simulink model "pcm_project"  (R2021b)
settings: Solver=VariableStepAuto  StartTime=0.0  StopTime=10  RelTol=1e-3
libraries: dspquant2 x2, dsparch4 x1, commutil2 x1, dspsigops x1
settings Model: Creator=ASUS i3  LastModifiedBy=ASUS i3
settings DataIOCC: SaveFormat=Array  SignalLoggingSaveFormat=ModelDataLogs  ReturnWorkspaceOutputs=off
settings OptimizationCC: BlockReduction=off  BooleanDataType=off
settings DebuggingCC: SaveWithParameterizedLinksMsg=none  UnderspecifiedInitializationDetection=Classic  MergeDetectMultiDrivingBlocksExec=none  SignalResolutionControl=TryResolveAllWithWarning  MultiTaskDSMMsg=warning  MultiTaskCondExecSysMsg=none  MultiTaskRateTransMsg=warning
settings HardwareCC: TargetUnknown=on
settings ModelReferenceCC: PropagateSignalLabelsOutOfModel=off
settings GRTTargetCC: CombineOutputUpdateFcns=off  GRTInterface=on

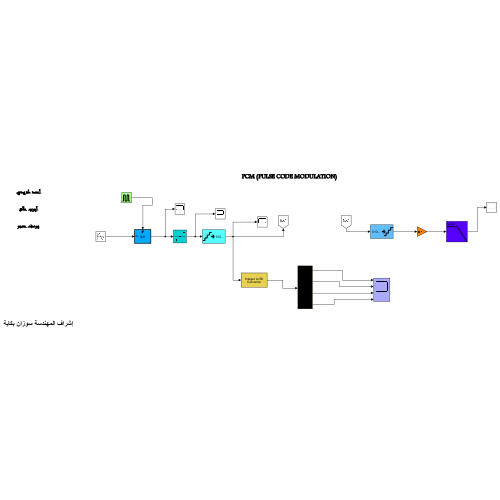
[thumbnail: Simulink's stored preview of the top-level diagram]
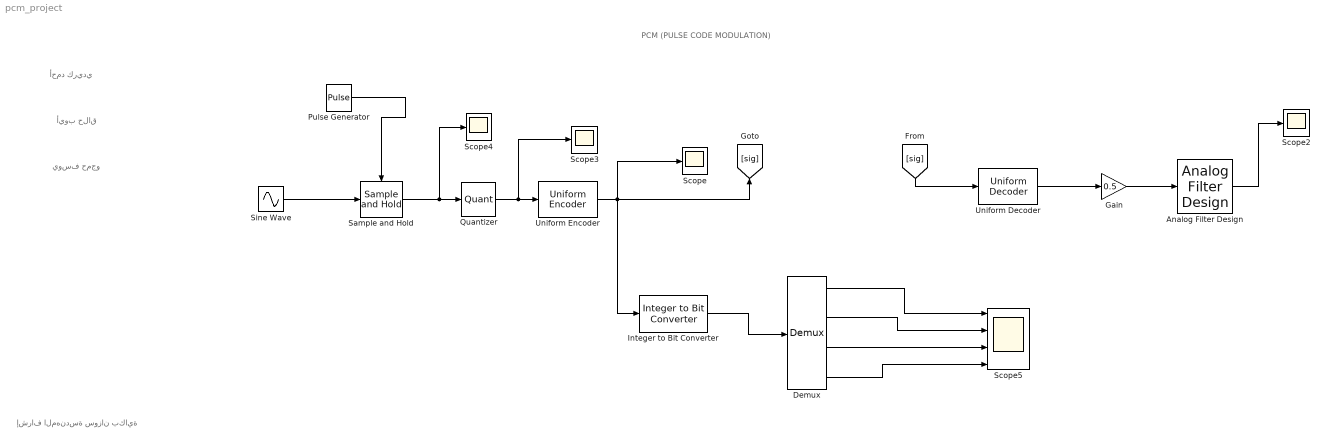
== system pcm_project ==
  note: يوسف حمجو
  note: أيوب حلاق
  note: أحمد كريدي
  note: إشراف المهندسة سوزان بكاية
  note: PCM (PULSE CODE MODULATION)
  Analog Filter Design : dsparch4/Analog Filter Design  method=Butterworth  filttype=Lowpass  N=8  Wlo=60  Whi=80  Rp=2  Rs=40
  Demux : Demux
  Gain : Gain  Gain=0.5
  Integer to Bit Converter : commutil2/Integer to Bit Converter  nbits=4  signedInputValues=Signed  bitOrder=MSB first  outDtype=Inherit via internal rule
  Pulse Generator : DiscretePulseGenerator  PulseType=Time based  Period=1/500  PulseWidth=5
  Quantizer : Quantizer  LinearizeAsGain=off
  Sample and Hold : dspsigops/Sample and Hold  trig=Rising edge  initCond=0  latchinput=off
  Scope{,2..4} (4 alike) : Scope
  Scope5 : Scope  NumInputPorts=4
  Sine Wave : Sin  Amplitude=5  Frequency=50  SampleTime=0
  Uniform Decoder : dspquant2/Uniform Decoder  peak=1  bits=3  overflowMode=Saturate  otype=Double
      settings: SourceProductBaseCode=DS
  Uniform Encoder : dspquant2/Uniform Encoder  peak=5  bits=4  otype=Signed integer
  wires:
  Sine Wave/1 -> Sample and Hold/1
  Sample and Hold/1 -> Scope4/1, Quantizer/1
  Uniform Encoder/1 -> Scope/1, [sig], Integer to Bit Converter/1
  Quantizer/1 -> Scope3/1, Uniform Encoder/1
  Integer to Bit Converter/1 -> Demux/1
  Demux/1 -> Scope5/1
  Demux/2 -> Scope5/2
  Demux/3 -> Scope5/3
  Demux/4 -> Scope5/4
  Uniform Decoder/1 -> Gain/1
  Gain/1 -> Analog Filter Design/1
  Analog Filter Design/1 -> Scope2/1
  Pulse Generator/1 -> Sample and Hold/Trigger
  [sig] -> Uniform Decoder/1
